simulink model "model2"  (R2023b)
settings: Solver=VariableStepAuto  StartTime=0.0  StopTime=8  RelTol=1e-3
values from neighbouring files (symbols this model uses):
  Bruitventx = 2    [dronecode.m]
  Bruitventy = 0.05    [dronecode.m]
  Consigneangle = pi/2    (= 1.570796327)    [dronecode.m]
  ConsigneVy = 0    [dronecode.m]
  Cx = 0.2    [dronecode.m]
  Freqfiltremoteur = 10    [dronecode.m]
  g = 9.81    [dronecode.m]
  J = 0.05    [dronecode.m]
  m = 0.9    [dronecode.m]
  pho = 1.225    [dronecode.m]
  Sref = 0.3    [dronecode.m]
libraries: simulink x9, cstblocks x3, embmathops x2, slpidlib x2, uavutilslib x1
settings Model: Creator=Utilisateur  LastModifiedBy=Utilisateur
settings SolverCC: ZeroCrossAlgorithm=Adaptive
settings OptimizationCC: ReuseModelBlockBuffer=off
settings DebuggingCC: IgnoredZcDiagnostic=none  UnconnectedInputMsg=warning  UnconnectedOutputMsg=warning  UnconnectedLineMsg=warning
settings ModelReferenceCC: EnableRefExpFcnMdlSchedulingChecks=on
settings RTWCC: DLArmComputeVersion=19.05

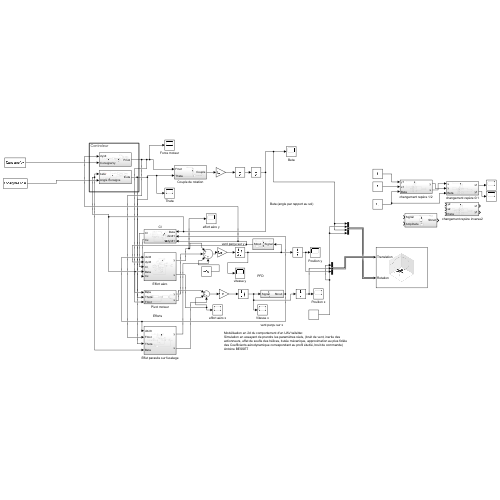
[thumbnail: Simulink's stored preview of the top-level diagram]
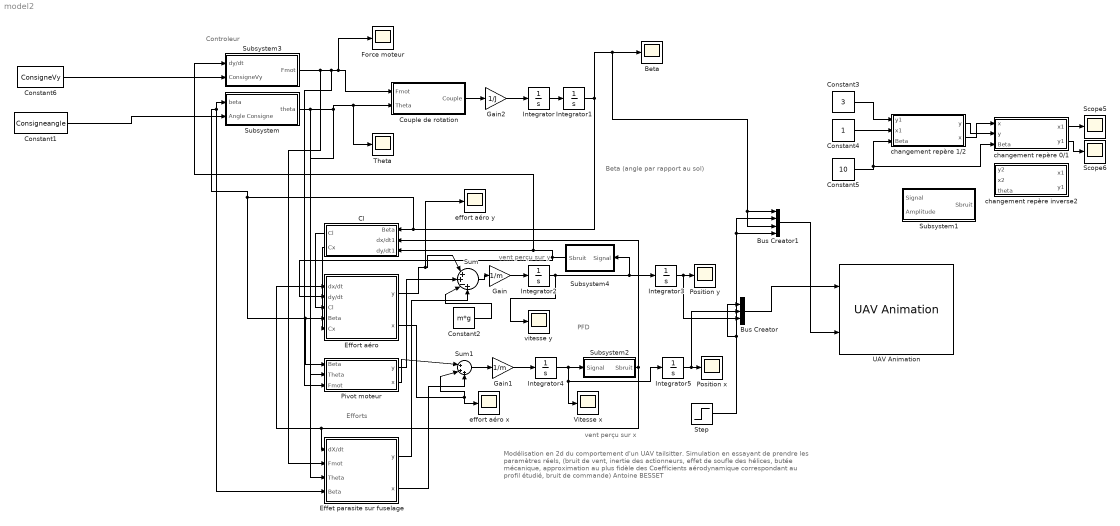
== system model2 ==
  note: vent perçu sur x
  note: Beta (angle par rapport au sol)
  note: Efforts
  note: PFD
  note: Controleur
  note: Modélisation en 2d du comportement d'un UAV tailsitter.
      | Simulation en essayant de prendre les paramètres réels, (bruit de vent, inertie des actionneurs, effet de soufle des hélices, butée mécanique, approximation au plus fidèle des Coefficients aérodynamique correspondant au profil étudié, bruit de commande)
      | Antoine BESSET
  note: vent perçu sur y
  Beta : Scope
  Bus Creator : BusCreator  Inputs=3
  Bus Creator1 : BusCreator  Inputs=4
  Cl : Subsystem
  Constant1 : Constant  Value=Consigneangle
  Constant2 : Constant  Value=m*g
  Constant3 : Constant  Value=3
  Constant4 : Constant
  Constant5 : Constant  Value=10
  Constant6 : Constant  Value=ConsigneVy
  Couple de rotation : Subsystem
  Effet parasite sur fuselage : Subsystem
  Effort aéro : Subsystem
  Force moteur : Scope
  Gain : Gain  Gain=1/m
  Gain1 : Gain  Gain=1/m
  Gain2 : Gain  Gain=1/J
  Integrator{,1,3,5} (4 alike) : Integrator
  Integrator2 : Integrator  LimitOutput=on  UpperSaturationLimit=100  LowerSaturationLimit=-100
  Integrator4 : Integrator  InitialCondition=10  LimitOutput=on  UpperSaturationLimit=100  LowerSaturationLimit=-100
  Pivot moteur : Subsystem
  Position x : Scope
  Position y : Scope
  Scope5 : Scope
  Scope6 : Scope
  Step : Step  Before=0.01  After=0.01  SampleTime=0
  Subsystem : Subsystem
  Subsystem1 : Subsystem
  Subsystem2 : Subsystem
  Subsystem3 : Subsystem
  Subsystem4 : Subsystem
  Sum : Sum  Inputs=|++-+
  Sum1 : Sum  Inputs=|+++
  Theta : Scope
  UAV Animation : uavutilslib/UAV Animation  UAVType=FixedWing  UAVSize=1  InertialZDirection=Up  SampleTime=-1
  Vitesse x : Scope
  changement repère 0/1 : Subsystem
  changement repère 1/2 : Subsystem
  changement repère inverse2 : Subsystem
  effort aéro x : Scope
  effort aéro y : Scope
  vitesse y : Scope
  wires:
  Subsystem/1(theta) -> Pivot moteur/2(Theta), Theta/1, Couple de rotation/2(Theta), Effet parasite sur fuselage/3(Theta)
  Integrator/1 -> Integrator1/1
  Cl/1(Cl) -> Effort aéro/3(Cl)
  Pivot moteur/1(y) -> Sum/2
  Constant2/1 -> Sum/3
  Pivot moteur/2(x) -> Sum1/1
  Effort aéro/2(x) -> effort aéro x/1, Sum1/2
  Gain1/1 -> Integrator4/1
  Sum1/1 -> Gain1/1
  Sum/1 -> Gain/1
  Gain/1 -> Integrator2/1
  Integrator4/1 -> Integrator5/1, Vitesse x/1, Subsystem2/1(Signal)
  Integrator5/1 -> Bus Creator/2, Position x/1
  Integrator2/1 -> Integrator3/1, Subsystem4/1(Signal), vitesse y/1
  Effort aéro/1(y) -> effort aéro y/1, Sum/1
  changement repère 1/2/2(x) -> changement repère 0/1/1(x)
  changement repère 1/2/1(y) -> changement repère 0/1/2(y)
  Constant5/1 -> changement repère 0/1/3(Beta), changement repère 1/2/3(Beta)
  Constant4/1 -> changement repère 1/2/2(x1)
  Constant3/1 -> changement repère 1/2/1(y1)
  changement repère 0/1/1(x1) -> Scope5/1
  changement repère 0/1/2(y1) -> Scope6/1
  Cl/2(Cx) -> Effort aéro/5(Cx)
  Couple de rotation/1(Couple) -> Gain2/1
  Gain2/1 -> Integrator/1
  Subsystem2/1(Sbruit) -> Cl/2(dx/dt1), Effet parasite sur fuselage/1(dX/dt), Effort aéro/1(dx/dt)
  Subsystem4/1(Sbruit) -> Subsystem3/1(dy/dt), Cl/3(dy/dt1), Effort aéro/2(dy/dt)
  Subsystem3/1(Fmot) -> Effet parasite sur fuselage/2(Fmot), Pivot moteur/3(Fmot), Force moteur/1, Couple de rotation/1(Fmot)
  Effet parasite sur fuselage/2(x) -> Sum1/3
  Effet parasite sur fuselage/1(y) -> Sum/4
  Constant6/1 -> Subsystem3/2(ConsigneVy)
  Constant1/1 -> Subsystem/2(Angle Consigne)
  Bus Creator/1 -> UAV Animation/1
  Step/1 -> Bus Creator1/4, Bus Creator1/2, Bus Creator/1
  Bus Creator1/1 -> UAV Animation/2
  Integrator3/1 -> Bus Creator/3, Position y/1
  Integrator1/1 -> Effet parasite sur fuselage/4(Beta), Subsystem/1(beta), Pivot moteur/1(Beta), Effort aéro/4(Beta), Cl/1(Beta), Bus Creator1/1, Bus Creator1/3, Beta/1

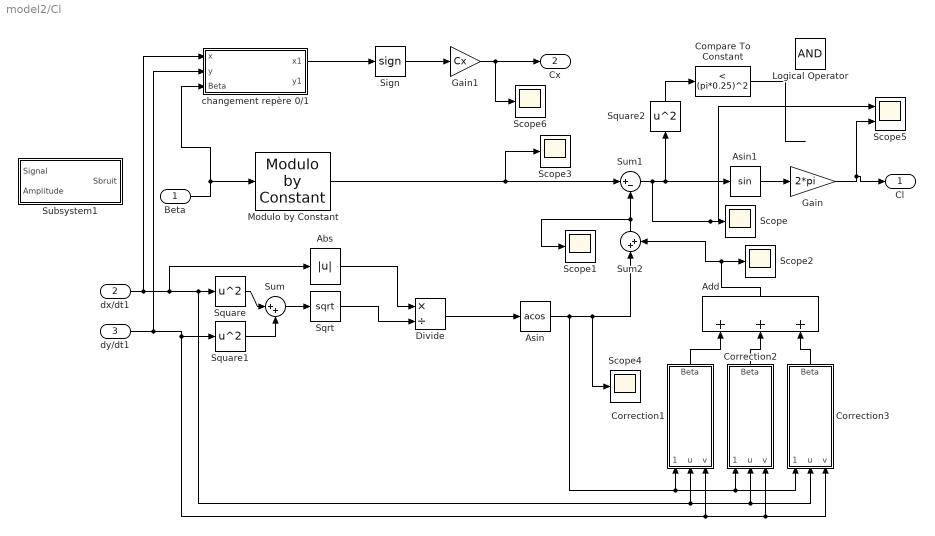
== system model2/Cl ==
  Beta : Inport
  dx/dt1 : Inport  Port=2
  dy/dt1 : Inport  Port=3
  Abs : Abs  SaturateOnIntegerOverflow=off
  Add : Sum  Inputs=+++
  Asin : Trigonometry  Operator=acos  OutputSignalType=real
  Asin1 : Trigonometry
  Compare To Constant : simulink/Logic and Bit Operations/Compare To Constant  relop=<  const=(pi*0.25)^2  OutDataTypeStr=boolean
  Correction1 : Subsystem
  Correction2 : Subsystem
  Correction3 : Subsystem
  Divide : Product  Inputs=*/
  Gain : Gain  Gain=2*pi
  Gain1 : Gain  Gain=Cx
  Logical Operator : Logic  AllPortsSameDT=off  OutDataTypeStr=boolean
  Modulo by Constant : embmathops/Modulo by Constant  Denominator=2*pi  SimulateUsing=Code generation
  Scope{,1..4,6} (6 alike) : Scope
  Scope5 : Scope  NumInputPorts=2
  Sign : Signum
  Sqrt : Sqrt
  Square : Math  Operator=square
  Square1 : Math  Operator=square
  Square2 : Math  Operator=square
  Subsystem1 : Subsystem
  Sum : Sum  Inputs=|++
  Sum1 : Sum  Inputs=|+-
  Sum2 : Sum  Inputs=|++
  changement repère 0/1 : Subsystem
  Cl : Outport
  Cx : Outport  Port=2
  wires:
  dy/dt1/1 -> changement repère 0/1/2(y), Correction3/3(v), Correction2/3(v), Correction1/3(v), Square1/1
  Square/1 -> Sum/1
  dx/dt1/1 -> changement repère 0/1/1(x), Correction3/2(u), Correction2/2(u), Correction1/2(u), Square/1, Abs/1
  Square1/1 -> Sum/2
  Sum/1 -> Sqrt/1
  Sqrt/1 -> Divide/2
  Divide/1 -> Asin/1
  Beta/1 -> changement repère 0/1/3(Beta), Modulo by Constant/1
  Modulo by Constant/1 -> Scope3/1, Sum1/1
  Abs/1 -> Divide/1
  Asin/1 -> Correction3/1(theta), Correction2/1(theta), Correction1/1(theta), Scope4/1, Sum2/1
  Add/1 -> Sum2/2, Scope2/1
  Correction1/1(Beta) -> Add/1
  Correction2/1(Beta) -> Add/2
  Correction3/1(Beta) -> Add/3
  Asin1/1 -> Gain/1
  Gain1/1 -> Scope6/1, Cx/1
  Sum2/1 -> Scope1/1, Sum1/2
  Sign/1 -> Gain1/1
  changement repère 0/1/1(x1) -> Sign/1
  Square2/1 -> Compare To Constant/1
  Gain/1 -> Scope5/2, Cl/1
  Compare To Constant/1 -> ?
  Sum1/1 -> Scope5/1, Scope/1, Asin1/1, Square2/1

== system model2/Couple de rotation ==
  Fmot : Inport
  Theta : Inport  Port=2
  Gain : Gain  Gain=0.10
  Product2 : Product
  Trigonometric Function : Trigonometry
  Couple : Outport
  wires:
  Theta/1 -> Trigonometric Function/1
  Fmot/1 -> Product2/2
  Trigonometric Function/1 -> Gain/1
  Product2/1 -> Couple/1
  Gain/1 -> Product2/1

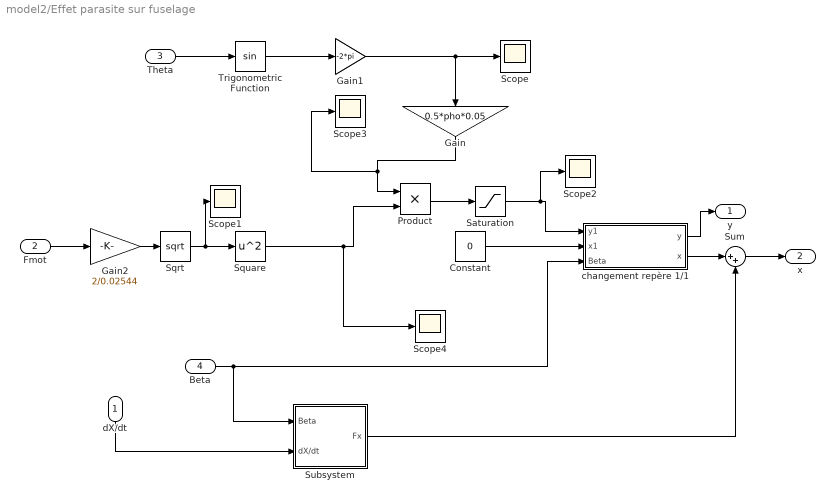
== system model2/Effet parasite sur fuselage ==
  dX/dt : Inport
  Fmot : Inport  Port=2
  Theta : Inport  Port=3
  Beta : Inport  Port=4
  Constant : Constant  Value=0
  Gain : Gain  Gain=0.5*pho*0.05
  Gain1 : Gain  Gain=-2*pi
  Gain2 : Gain  Gain=2/0.02544
  Product : Product
  Saturation : Saturate  UpperLimit=20  LowerLimit=-20
  Scope{,1..4} (5 alike) : Scope
  Sqrt : Sqrt
  Square : Math  Operator=square
  Subsystem : Subsystem
  Sum : Sum  Inputs=|++
  Trigonometric Function : Trigonometry
  changement repère 1/1 : Subsystem
  y : Outport
  x : Outport  Port=2
  wires:
  Square/1 -> Scope4/1, Product/2
  Gain/1 -> Scope3/1, Product/1
  Beta/1 -> Subsystem/1(Beta), changement repère 1/1/3(Beta)
  changement repère 1/1/1(y) -> y/1
  Gain1/1 -> Scope/1, Gain/1
  Gain2/1 -> Sqrt/1
  Fmot/1 -> Gain2/1
  Sqrt/1 -> Scope1/1, Square/1
  Constant/1 -> changement repère 1/1/2(x1)
  Theta/1 -> Trigonometric Function/1
  Trigonometric Function/1 -> Gain1/1
  Product/1 -> Saturation/1
  Saturation/1 -> Scope2/1, changement repère 1/1/1(y1)
  dX/dt/1 -> Subsystem/2(dX/dt)
  changement repère 1/1/2(x) -> Sum/1
  Sum/1 -> x/1
  Subsystem/1(Fx) -> Sum/2

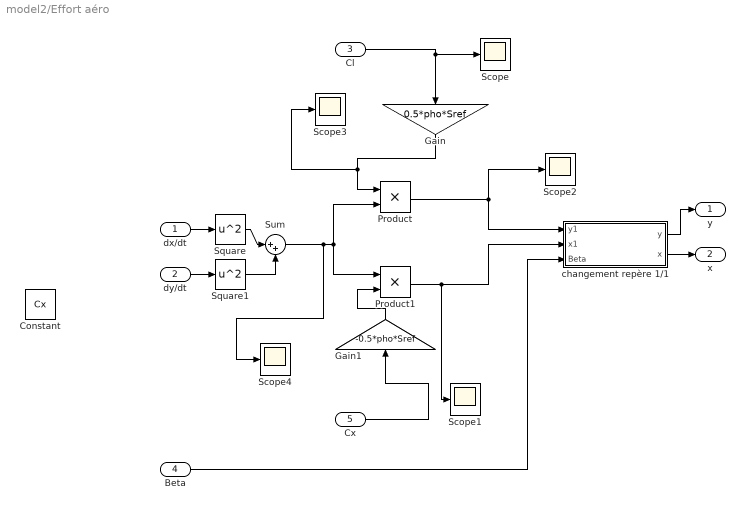
== system model2/Effort aéro ==
  dx/dt : Inport
  dy/dt : Inport  Port=2
  Cl : Inport  Port=3
  Beta : Inport  Port=4
  Cx : Inport  Port=5
  Constant : Constant  Value=Cx
  Gain : Gain  Gain=0.5*pho*Sref
  Gain1 : Gain  Gain=-0.5*pho*Sref
  Product : Product
  Product1 : Product
  Scope{,1..4} (5 alike) : Scope
  Square : Math  Operator=square
  Square1 : Math  Operator=square
  Sum : Sum  Inputs=|++
  changement repère 1/1 : Subsystem
  y : Outport
  x : Outport  Port=2
  wires:
  dx/dt/1 -> Square/1
  dy/dt/1 -> Square1/1
  Square1/1 -> Sum/2
  Square/1 -> Sum/1
  Sum/1 -> Scope4/1, Product1/1, Product/2
  Cl/1 -> Scope/1, Gain/1
  Gain/1 -> Scope3/1, Product/1
  Gain1/1 -> Product1/2
  Product/1 -> changement repère 1/1/1(y1), Scope2/1
  Product1/1 -> Scope1/1, changement repère 1/1/2(x1)
  Beta/1 -> changement repère 1/1/3(Beta)
  changement repère 1/1/2(x) -> x/1
  changement repère 1/1/1(y) -> y/1
  Cx/1 -> Gain1/1

== system model2/Pivot moteur ==
  Beta : Inport
  Theta : Inport  Port=2
  Fmot : Inport  Port=3
  Constant : Constant  Value=0
  changement repère 1/1 : Subsystem
  changement repère inverse2/1 : Subsystem
  y : Outport
  x : Outport  Port=2
  wires:
  Theta/1 -> changement repère inverse2/1/3(theta)
  Fmot/1 -> changement repère inverse2/1/2(x2)
  changement repère inverse2/1/2(y1) -> changement repère 1/1/1(y1)
  changement repère inverse2/1/1(x1) -> changement repère 1/1/2(x1)
  changement repère 1/1/2(x) -> x/1
  changement repère 1/1/1(y) -> y/1
  Constant/1 -> changement repère inverse2/1/1(y2)
  Beta/1 -> changement repère 1/1/3(Beta)

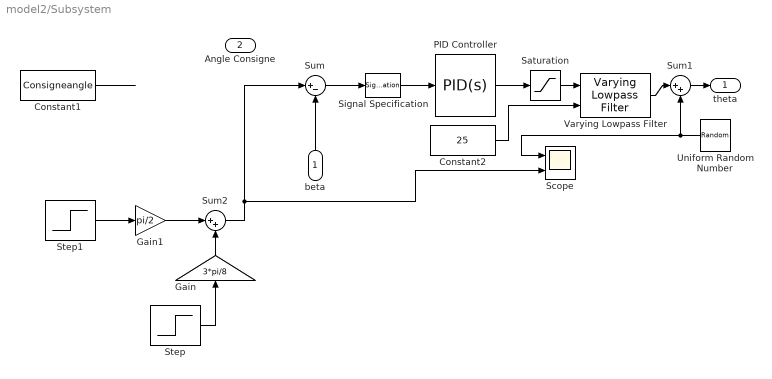
== system model2/Subsystem ==
  beta : Inport
  Angle Consigne : Inport  Port=2
  Constant1 : Constant  Value=Consigneangle
  Constant2 : Constant  Value=25
  Gain : Gain  Gain=3*pi/8
  Gain1 : Gain  Gain=pi/2
  PID Controller : slpidlib/PID Controller  Controller=PID  Form=Parallel  TimeDomain=Continuous-time  UseExternalTs=off  SampleTime=-1  IntegratorMethod=Forward Euler  FilterMethod=Forward Euler  ControllerParametersSource=internal  P=1  I=0.3  UseKiTs=off  D=0.5  N=100  UseFilter=on  TunerSelectOption=Transfer Function Based (PID Tuner App)  InitialConditionSource=internal  InitialConditionForIntegrator=0  InitialConditionForFilter=0  DifferentiatorICPrevScaledInput=0  ExternalReset=none  TrackingMode=off  Kt=1  LimitOutput=on  SatLimitsSource=internal  UpperSaturationLimit=pi/4  LowerSaturationLimit=-pi/4  LinearizeAsGain=on  AntiWindupMode=none  Kb=1  LimitIntegrator=off  UpperIntegratorSaturationLimit=inf  LowerIntegratorSaturationLimit=-inf  POutMin=[]  POutMax=[]  IOutMin=[]  IOutMax=[]  DOutMin=[]  DOutMax=[]  NOutMin=[]  NOutMax=[]  SumOutMin=[]  SumOutMax=[]  SaturationOutMin=[]  SaturationOutMax=[]  PParamMin=[]  PParamMax=[]  IParamMin=[]  IParamMax=[]  DParamMin=[]  DParamMax=[]  NParamMin=[]  NParamMax=[]  KbParamMin=[]  KbParamMax=[]  KtParamMin=[]  KtParamMax=[]  KbOutMin=[]  KbOutMax=[]  KtOutMin=[]  KtOutMax=[]  IntegratorOutMin=[]  IntegratorOutMax=[]  FilterOutMin=[]  FilterOutMax=[]  SumI1OutMin=[]  SumI1OutMax=[]  SumI2OutMin=[]  SumI2OutMax=[]  SumI3OutMin=[]  SumI3OutMax=[]  SumI4OutMin=[]  SumI4OutMax=[]  SumDOutMin=[]  SumDOutMax=[]  DifferentiatorOutMin=[]  DifferentiatorOutMax=[]  FilterDiffOutCoefMin=[]  FilterDiffOutCoefMax=[]  ReciprocalOutMin=[]  ReciprocalOutMax=[]  SumDenOutMin=[]  SumDenOutMax=[]  SumNumOutMin=[]  SumNumOutMax=[]  DivideOutMin=[]  DivideOutMax=[]  UdiffTsProdOutMin=[]  UdiffTsProdOutMax=[]  NTsProdOutMin=[]  NTsProdOutMax=[]  UintegralTsProdOutMin=[]  UintegralTsProdOutMax=[]  UngainTsProdOutMin=[]  UngainTsProdOutMax=[]  ClampingZeroOutDataTypeStr=Inherit: Inherit via back propagation  ClampingZeroOutMin=[]  ClampingZeroOutMax=[]  FilterDenConstantOutDataTypeStr=Inherit: Inherit via back propagation  FilterDenConstantOutMin=[]  FilterDenConstantOutMax=[]  PCopyOutDataTypeStr=Inherit: Inherit via back propagation  PCopyOutMin=[]  PCopyOutMax=[]  NCopyOutDataTypeStr=Inherit: Inherit via back propagation  NCopyOutMin=[]  NCopyOutMax=[]  IntegratorContinuousStateAttributes=''  IntegratorStateMustResolveToSignalObject=off  IntegratorRTWStateStorageClass=Auto  FilterContinuousStateAttributes=''  FilterStateMustResolveToSignalObject=off  FilterRTWStateStorageClass=Auto  ParallelPVariant=InternalParameters  IdealPVariant=Disabled  IVariant=InternalParameters  DVariant=InternalParameters  IntegratorVariant=Continuous  SatVariant=Enabled  AWVariant=Passthrough  PCopyVariant=Disabled  TRVariant=Disabled  FdbkBlocksVariant=Forward  IdealPFdbkVariant=Disabled  SatFdbkVariant=Disabled  DerivativeFilterVariant=ContFilter  NVariant=InternalParameters  NCopyVariant=Disabled  FilterICVariant=InternalICsFilter  IntegratorICVariant=InternalICs  ExternalResetVariant=Disabled  TRSumVariant=Passthrough  SumFdbkVariant=Disabled  SumVariant=Sum_PID  TsampFilterVariant=InternalTs  TsampNgainVariant=Passthrough  TsampIntegralVariant=Disabled_SignalSpec  ExternalSaturationOutDataTypeStr=Inherit: Same as second input
  Saturation : Saturate  UpperLimit=pi/4  LowerLimit=-pi/4
  Scope : Scope  NumInputPorts=2
  Signal Specification : SignalSpecification  Dimensions=1
  Step : Step  Time=5  After=-1  SampleTime=0
  Step1 : Step  Before=0.1  SampleTime=0
  Sum : Sum  Inputs=|+-
  Sum1 : Sum  Inputs=|++
  Sum2 : Sum  Inputs=|++
  Uniform Random Number : UniformRandomNumber  Minimum=-0.05  Maximum=0.05  SampleTime=0.01
  Varying Lowpass Filter : cstblocks/Linear Parameter Varying/Varying Lowpass Filter  N=1
  theta : Outport
  wires:
  beta/1 -> Sum/2
  Sum1/1 -> theta/1
  Uniform Random Number/1 -> Scope/1, Sum1/2
  Signal Specification/1 -> PID Controller/1
  Sum/1 -> Signal Specification/1
  Gain/1 -> Sum2/2
  Step/1 -> Gain/1
  Gain1/1 -> Sum2/1
  Step1/1 -> Gain1/1
  PID Controller/1 -> Saturation/1
  Saturation/1 -> Varying Lowpass Filter/1
  Varying Lowpass Filter/1 -> Sum1/1
  Constant2/1 -> Varying Lowpass Filter/2
  Constant1/1 -> ?
  Sum2/1 -> Sum/1, Scope/2

== system model2/Subsystem1 ==
  Signal : Inport
  Amplitude : Inport  Port=2
  Product : Product
  Sum2 : Sum  Inputs=|++
  Uniform Random Number : UniformRandomNumber  SampleTime=0.01
  Sbruit : Outport
  wires:
  Signal/1 -> Sum2/1
  Sum2/1 -> Sbruit/1
  Uniform Random Number/1 -> Product/2
  Product/1 -> Sum2/2
  Amplitude/1 -> Product/1

== system model2/Subsystem2 ==
  Signal : Inport
  Constant : Constant  Value=Bruitventx
  Constant2 : Constant
  Product : Product
  Scope : Scope
  Sum2 : Sum  Inputs=|++
  Uniform Random Number : UniformRandomNumber  Minimum=-10  Maximum=10  SampleTime=0.01
  Varying Lowpass Filter1 : cstblocks/Linear Parameter Varying/Varying Lowpass Filter  N=1
  Sbruit : Outport
  wires:
  Signal/1 -> Sum2/1
  Uniform Random Number/1 -> Product/2
  Constant/1 -> Product/1
  Sum2/1 -> Sbruit/1
  Constant2/1 -> Varying Lowpass Filter1/2
  Product/1 -> Varying Lowpass Filter1/1
  Varying Lowpass Filter1/1 -> Scope/1, Sum2/2

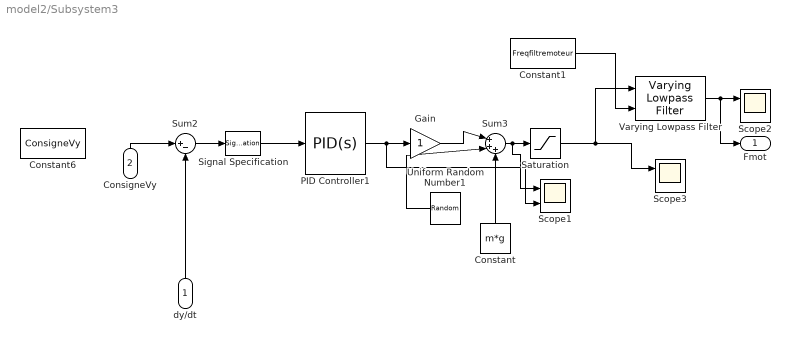
== system model2/Subsystem3 ==
  dy/dt : Inport
  ConsigneVy : Inport  Port=2
  Constant : Constant  Value=m*g
  Constant1 : Constant  Value=Freqfiltremoteur
  Constant6 : Constant  Value=ConsigneVy
  Gain : Gain
  PID Controller1 : slpidlib/PID Controller  Controller=PID  Form=Parallel  TimeDomain=Continuous-time  UseExternalTs=off  SampleTime=0.1  IntegratorMethod=Forward Euler  FilterMethod=Forward Euler  ControllerParametersSource=internal  P=1.2  I=0.6  UseKiTs=off  D=0.2  N=100  UseFilter=on  TunerSelectOption=Transfer Function Based (PID Tuner App)  InitialConditionSource=internal  InitialConditionForIntegrator=0  InitialConditionForFilter=0  DifferentiatorICPrevScaledInput=0  ExternalReset=none  TrackingMode=off  Kt=1  LimitOutput=off  SatLimitsSource=internal  UpperSaturationLimit=inf  LowerSaturationLimit=-inf  LinearizeAsGain=on  AntiWindupMode=none  Kb=1  LimitIntegrator=off  UpperIntegratorSaturationLimit=inf  LowerIntegratorSaturationLimit=-inf  POutMin=[]  POutMax=[]  IOutMin=[]  IOutMax=[]  DOutMin=[]  DOutMax=[]  NOutMin=[]  NOutMax=[]  SumOutMin=[]  SumOutMax=[]  SaturationOutMin=[]  SaturationOutMax=[]  PParamMin=[]  PParamMax=[]  IParamMin=[]  IParamMax=[]  DParamMin=[]  DParamMax=[]  NParamMin=[]  NParamMax=[]  KbParamMin=[]  KbParamMax=[]  KtParamMin=[]  KtParamMax=[]  KbOutMin=[]  KbOutMax=[]  KtOutMin=[]  KtOutMax=[]  IntegratorOutMin=[]  IntegratorOutMax=[]  FilterOutMin=[]  FilterOutMax=[]  SumI1OutMin=[]  SumI1OutMax=[]  SumI2OutMin=[]  SumI2OutMax=[]  SumI3OutMin=[]  SumI3OutMax=[]  SumI4OutMin=[]  SumI4OutMax=[]  SumDOutMin=[]  SumDOutMax=[]  DifferentiatorOutMin=[]  DifferentiatorOutMax=[]  FilterDiffOutCoefMin=[]  FilterDiffOutCoefMax=[]  ReciprocalOutMin=[]  ReciprocalOutMax=[]  SumDenOutMin=[]  SumDenOutMax=[]  SumNumOutMin=[]  SumNumOutMax=[]  DivideOutMin=[]  DivideOutMax=[]  UdiffTsProdOutMin=[]  UdiffTsProdOutMax=[]  NTsProdOutMin=[]  NTsProdOutMax=[]  UintegralTsProdOutMin=[]  UintegralTsProdOutMax=[]  UngainTsProdOutMin=[]  UngainTsProdOutMax=[]  ClampingZeroOutDataTypeStr=Inherit: Inherit via back propagation  ClampingZeroOutMin=[]  ClampingZeroOutMax=[]  FilterDenConstantOutDataTypeStr=Inherit: Inherit via back propagation  FilterDenConstantOutMin=[]  FilterDenConstantOutMax=[]  PCopyOutDataTypeStr=Inherit: Inherit via back propagation  PCopyOutMin=[]  PCopyOutMax=[]  NCopyOutDataTypeStr=Inherit: Inherit via back propagation  NCopyOutMin=[]  NCopyOutMax=[]  IntegratorContinuousStateAttributes=''  IntegratorStateMustResolveToSignalObject=off  IntegratorRTWStateStorageClass=Auto  FilterContinuousStateAttributes=''  FilterStateMustResolveToSignalObject=off  FilterRTWStateStorageClass=Auto  ParallelPVariant=InternalParameters  IdealPVariant=Disabled  IVariant=InternalParameters  DVariant=InternalParameters  IntegratorVariant=Continuous  SatVariant=Disabled  AWVariant=Passthrough  PCopyVariant=Disabled  TRVariant=Disabled  FdbkBlocksVariant=Forward  IdealPFdbkVariant=Disabled  SatFdbkVariant=Disabled  DerivativeFilterVariant=ContFilter  NVariant=InternalParameters  NCopyVariant=Disabled  FilterICVariant=InternalICsFilter  IntegratorICVariant=InternalICs  ExternalResetVariant=Disabled  TRSumVariant=Passthrough  SumFdbkVariant=Disabled  SumVariant=Sum_PID  TsampFilterVariant=InternalTs  TsampNgainVariant=Passthrough  TsampIntegralVariant=Disabled_SignalSpec  ExternalSaturationOutDataTypeStr=Inherit: Same as second input
  Saturation : Saturate  UpperLimit=40  LowerLimit=0
  Scope1 : Scope  NumInputPorts=2
  Scope2 : Scope  NumInputPorts=2
  Scope3 : Scope  NumInputPorts=2
  Signal Specification : SignalSpecification  Dimensions=1
  Sum2 : Sum  Inputs=|+-
  Sum3 : Sum  Inputs=|+++
  Uniform Random Number1 : UniformRandomNumber  Minimum=-0.01  Maximum=0.01  SampleTime=0.01
  Varying Lowpass Filter : cstblocks/Linear Parameter Varying/Varying Lowpass Filter  N=1
  Fmot : Outport
  wires:
  Saturation/1 -> Varying Lowpass Filter/1, Scope3/1
  dy/dt/1 -> Sum2/2
  Sum3/1 -> Scope1/1, Saturation/1
  Uniform Random Number1/1 -> Sum3/2
  PID Controller1/1 -> Gain/1, Scope1/2
  Constant/1 -> Sum3/3
  Gain/1 -> Sum3/1
  Sum2/1 -> Signal Specification/1
  Signal Specification/1 -> PID Controller1/1
  Varying Lowpass Filter/1 -> Fmot/1, Scope2/1
  Constant1/1 -> Varying Lowpass Filter/2
  ConsigneVy/1 -> Sum2/1

== system model2/Subsystem4 ==
  Signal : Inport
  Constant1 : Constant  Value=Bruitventy
  Product : Product
  Sum2 : Sum  Inputs=|++
  Uniform Random Number : UniformRandomNumber  SampleTime=0.01
  Sbruit : Outport
  wires:
  Signal/1 -> Sum2/1
  Sum2/1 -> Sbruit/1
  Uniform Random Number/1 -> Product/2
  Product/1 -> Sum2/2
  Constant1/1 -> Product/1

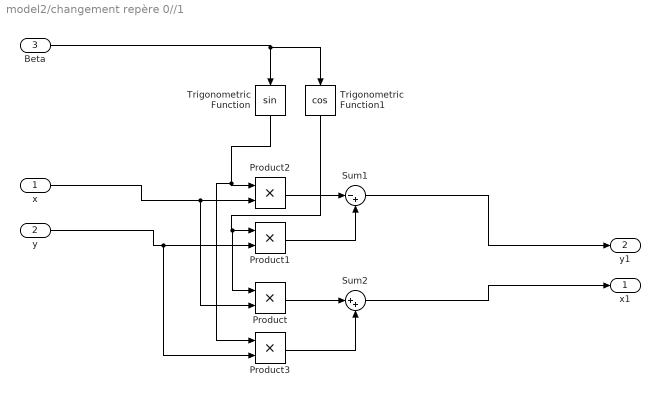
== system model2/changement repère 0//1 ==
  x : Inport
  y : Inport  Port=2
  Beta : Inport  Port=3
  Product{,1..3} (4 alike) : Product
  Sum1 : Sum  Inputs=|-+
  Sum2 : Sum  Inputs=|++
  Trigonometric Function : Trigonometry
  Trigonometric Function1 : Trigonometry  Operator=cos
  x1 : Outport
  y1 : Outport  Port=2
  wires:
  Beta/1 -> Trigonometric Function1/1, Trigonometric Function/1
  Trigonometric Function/1 -> Product3/1, Product2/1
  Product2/1 -> Sum1/1
  x/1 -> Product/2, Product2/2
  y/1 -> Product3/2, Product1/2
  Trigonometric Function1/1 -> Product/1, Product1/1
  Product1/1 -> Sum1/2
  Sum1/1 -> y1/1
  Product3/1 -> Sum2/2
  Product/1 -> Sum2/1
  Sum2/1 -> x1/1

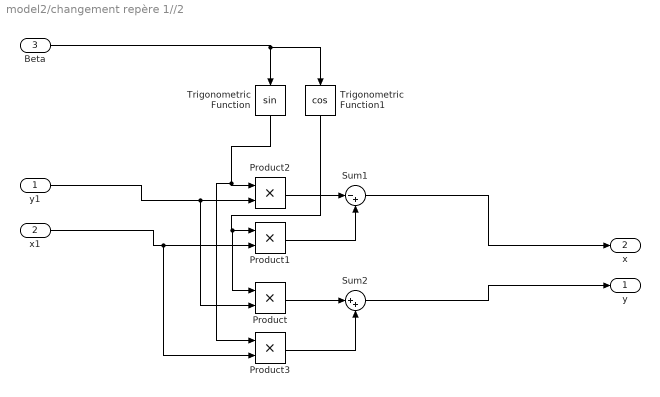
== system model2/changement repère 1//2 ==
  y1 : Inport
  x1 : Inport  Port=2
  Beta : Inport  Port=3
  Product{,1..3} (4 alike) : Product
  Sum1 : Sum  Inputs=|-+
  Sum2 : Sum  Inputs=|++
  Trigonometric Function : Trigonometry
  Trigonometric Function1 : Trigonometry  Operator=cos
  y : Outport
  x : Outport  Port=2
  wires:
  Beta/1 -> Trigonometric Function1/1, Trigonometric Function/1
  Trigonometric Function/1 -> Product3/1, Product2/1
  Product2/1 -> Sum1/1
  y1/1 -> Product/2, Product2/2
  x1/1 -> Product3/2, Product1/2
  Trigonometric Function1/1 -> Product/1, Product1/1
  Product1/1 -> Sum1/2
  Sum1/1 -> x/1
  Product3/1 -> Sum2/2
  Product/1 -> Sum2/1
  Sum2/1 -> y/1

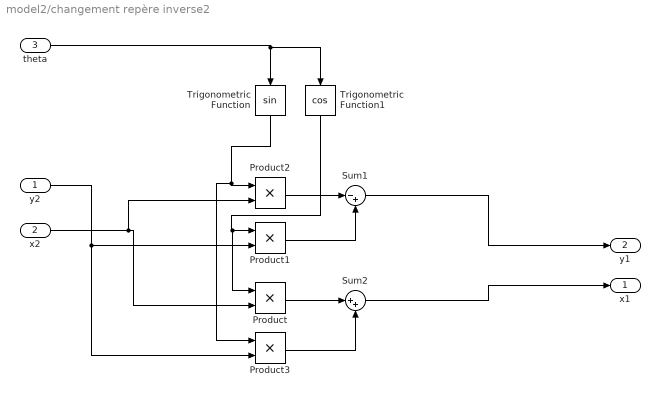
== system model2/changement repère inverse2 ==
  y2 : Inport
  x2 : Inport  Port=2
  theta : Inport  Port=3
  Product{,1..3} (4 alike) : Product
  Sum1 : Sum  Inputs=|-+
  Sum2 : Sum  Inputs=|++
  Trigonometric Function : Trigonometry
  Trigonometric Function1 : Trigonometry  Operator=cos
  x1 : Outport
  y1 : Outport  Port=2
  wires:
  theta/1 -> Trigonometric Function1/1, Trigonometric Function/1
  Trigonometric Function/1 -> Product3/1, Product2/1
  Product2/1 -> Sum1/1
  Trigonometric Function1/1 -> Product/1, Product1/1
  Product1/1 -> Sum1/2
  Sum1/1 -> y1/1
  Product3/1 -> Sum2/2
  Product/1 -> Sum2/1
  Sum2/1 -> x1/1
  x2/1 -> Product2/2, Product/2
  y2/1 -> Product1/2, Product3/2

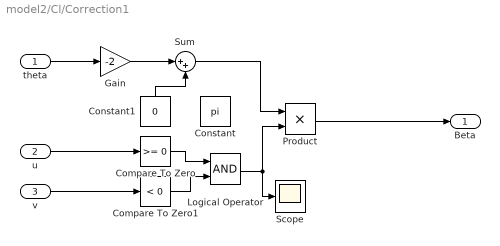
== system model2/Cl/Correction1 ==
  theta : Inport
  u : Inport  Port=2
  v : Inport  Port=3
  Compare To Zero : simulink/Logic and Bit Operations/Compare To Zero  relop=>=  OutDataTypeStr=boolean
  Compare To Zero1 : simulink/Logic and Bit Operations/Compare To Zero  relop=<  OutDataTypeStr=boolean
  Constant : Constant  Value=pi
  Constant1 : Constant  Value=0
  Gain : Gain  Gain=-2
  Logical Operator : Logic  AllPortsSameDT=off  OutDataTypeStr=boolean
  Product : Product
  Scope : Scope
  Sum : Sum  Inputs=|++
  Beta : Outport
  wires:
  u/1 -> Compare To Zero/1
  v/1 -> Compare To Zero1/1
  Compare To Zero/1 -> Logical Operator/1
  Compare To Zero1/1 -> Logical Operator/2
  Product/1 -> Beta/1
  Sum/1 -> Product/1
  theta/1 -> Gain/1
  Gain/1 -> Sum/1
  Constant1/1 -> Sum/2
  Logical Operator/1 -> Product/2, Scope/1

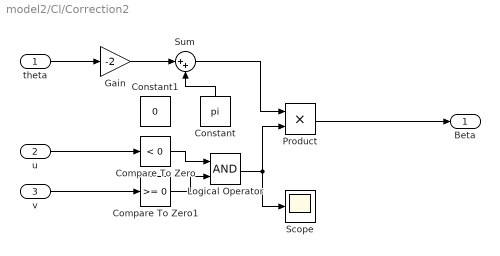
== system model2/Cl/Correction2 ==
  theta : Inport
  u : Inport  Port=2
  v : Inport  Port=3
  Compare To Zero : simulink/Logic and Bit Operations/Compare To Zero  relop=<  OutDataTypeStr=boolean
  Compare To Zero1 : simulink/Logic and Bit Operations/Compare To Zero  relop=>=  OutDataTypeStr=boolean
  Constant : Constant  Value=pi
  Constant1 : Constant  Value=0
  Gain : Gain  Gain=-2
  Logical Operator : Logic  AllPortsSameDT=off  OutDataTypeStr=boolean
  Product : Product
  Scope : Scope
  Sum : Sum  Inputs=|++
  Beta : Outport
  wires:
  u/1 -> Compare To Zero/1
  v/1 -> Compare To Zero1/1
  Compare To Zero/1 -> Logical Operator/1
  Compare To Zero1/1 -> Logical Operator/2
  Logical Operator/1 -> Product/2, Scope/1
  Product/1 -> Beta/1
  Sum/1 -> Product/1
  theta/1 -> Gain/1
  Gain/1 -> Sum/1
  Constant/1 -> Sum/2

== system model2/Cl/Correction3 ==
  theta : Inport
  u : Inport  Port=2
  v : Inport  Port=3
  Compare To Zero : simulink/Logic and Bit Operations/Compare To Zero  relop=<  OutDataTypeStr=boolean
  Compare To Zero1 : simulink/Logic and Bit Operations/Compare To Zero  relop=<  OutDataTypeStr=boolean
  Constant : Constant  Value=pi
  Constant1 : Constant  Value=0
  Gain : Gain  Gain=0
  Logical Operator : Logic  AllPortsSameDT=off  OutDataTypeStr=boolean
  Product : Product
  Scope : Scope
  Sum : Sum  Inputs=|++
  Beta : Outport
  wires:
  u/1 -> Compare To Zero/1
  v/1 -> Compare To Zero1/1
  Compare To Zero/1 -> Logical Operator/1
  Compare To Zero1/1 -> Logical Operator/2
  Logical Operator/1 -> Product/2, Scope/1
  Product/1 -> Beta/1
  Sum/1 -> Product/1
  theta/1 -> Gain/1
  Gain/1 -> Sum/1
  Constant/1 -> Sum/2

== system model2/Cl/Subsystem1 ==
  Signal : Inport
  Amplitude : Inport  Port=2
  Product : Product
  Sum2 : Sum  Inputs=|++
  Uniform Random Number : UniformRandomNumber  SampleTime=0.01
  Sbruit : Outport
  wires:
  Signal/1 -> Sum2/1
  Sum2/1 -> Sbruit/1
  Uniform Random Number/1 -> Product/2
  Product/1 -> Sum2/2
  Amplitude/1 -> Product/1

== system model2/Cl/changement repère 0//1 ==
  x : Inport
  y : Inport  Port=2
  Beta : Inport  Port=3
  Product{,1..3} (4 alike) : Product
  Sum1 : Sum  Inputs=|-+
  Sum2 : Sum  Inputs=|++
  Trigonometric Function : Trigonometry
  Trigonometric Function1 : Trigonometry  Operator=cos
  x1 : Outport
  y1 : Outport  Port=2
  wires:
  Beta/1 -> Trigonometric Function1/1, Trigonometric Function/1
  Trigonometric Function/1 -> Product3/1, Product2/1
  Product2/1 -> Sum1/1
  x/1 -> Product/2, Product2/2
  y/1 -> Product3/2, Product1/2
  Trigonometric Function1/1 -> Product/1, Product1/1
  Product1/1 -> Sum1/2
  Sum1/1 -> y1/1
  Product3/1 -> Sum2/2
  Product/1 -> Sum2/1
  Sum2/1 -> x1/1

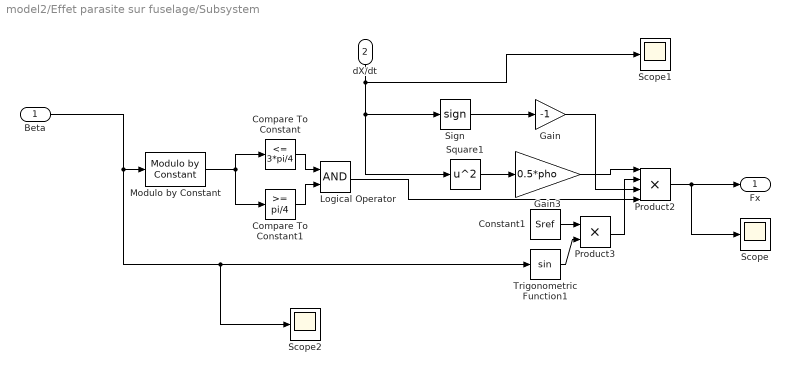
== system model2/Effet parasite sur fuselage/Subsystem ==
  Beta : Inport
  dX/dt : Inport  Port=2
  Compare To Constant : simulink/Logic and Bit Operations/Compare To Constant  relop=<=  const=3*pi/4  OutDataTypeStr=boolean
  Compare To Constant1 : simulink/Logic and Bit Operations/Compare To Constant  relop=>=  const=pi/4  OutDataTypeStr=boolean
  Constant1 : Constant  Value=Sref
  Gain : Gain  Gain=-1
  Gain3 : Gain  Gain=0.5*pho
  Logical Operator : Logic  AllPortsSameDT=off  OutDataTypeStr=boolean
  Modulo by Constant : embmathops/Modulo by Constant  Denominator=2*pi  SimulateUsing=Code generation
  Product2 : Product  Inputs=4
  Product3 : Product
  Scope : Scope
  Scope1 : Scope
  Scope2 : Scope
  Sign : Signum
  Square1 : Math  Operator=square
  Trigonometric Function1 : Trigonometry
  Fx : Outport
  wires:
  Beta/1 -> Scope2/1, Trigonometric Function1/1, Modulo by Constant/1
  Product3/1 -> Product2/2
  Compare To Constant1/1 -> Logical Operator/2
  Compare To Constant/1 -> Logical Operator/1
  Gain3/1 -> Product2/1
  Trigonometric Function1/1 -> Product3/2
  Square1/1 -> Gain3/1
  Modulo by Constant/1 -> Compare To Constant1/1, Compare To Constant/1
  dX/dt/1 -> Square1/1, Sign/1, Scope1/1
  Product2/1 -> Scope/1, Fx/1
  Constant1/1 -> Product3/1
  Sign/1 -> Gain/1
  Gain/1 -> Product2/3
  Logical Operator/1 -> Product2/4

== system model2/Effet parasite sur fuselage/changement repère 1//1 ==
  y1 : Inport
  x1 : Inport  Port=2
  Beta : Inport  Port=3
  Product{,1..3} (4 alike) : Product
  Sum1 : Sum  Inputs=|-+
  Sum2 : Sum  Inputs=|++
  Trigonometric Function : Trigonometry
  Trigonometric Function1 : Trigonometry  Operator=cos
  y : Outport
  x : Outport  Port=2
  wires:
  Beta/1 -> Trigonometric Function1/1, Trigonometric Function/1
  Trigonometric Function/1 -> Product3/1, Product2/1
  Product2/1 -> Sum1/1
  y1/1 -> Product/2, Product2/2
  x1/1 -> Product3/2, Product1/2
  Trigonometric Function1/1 -> Product/1, Product1/1
  Product1/1 -> Sum1/2
  Sum1/1 -> x/1
  Product3/1 -> Sum2/2
  Product/1 -> Sum2/1
  Sum2/1 -> y/1

== system model2/Effort aéro/changement repère 1//1 ==
  y1 : Inport
  x1 : Inport  Port=2
  Beta : Inport  Port=3
  Product{,1..3} (4 alike) : Product
  Sum1 : Sum  Inputs=|-+
  Sum2 : Sum  Inputs=|++
  Trigonometric Function : Trigonometry
  Trigonometric Function1 : Trigonometry  Operator=cos
  y : Outport
  x : Outport  Port=2
  wires:
  Beta/1 -> Trigonometric Function1/1, Trigonometric Function/1
  Trigonometric Function/1 -> Product3/1, Product2/1
  Product2/1 -> Sum1/1
  y1/1 -> Product/2, Product2/2
  x1/1 -> Product3/2, Product1/2
  Trigonometric Function1/1 -> Product/1, Product1/1
  Product1/1 -> Sum1/2
  Sum1/1 -> x/1
  Product3/1 -> Sum2/2
  Product/1 -> Sum2/1
  Sum2/1 -> y/1

== system model2/Pivot moteur/changement repère 1//1 ==
  y1 : Inport
  x1 : Inport  Port=2
  Beta : Inport  Port=3
  Product{,1..3} (4 alike) : Product
  Sum1 : Sum  Inputs=|-+
  Sum2 : Sum  Inputs=|++
  Trigonometric Function : Trigonometry
  Trigonometric Function1 : Trigonometry  Operator=cos
  y : Outport
  x : Outport  Port=2
  wires:
  Beta/1 -> Trigonometric Function1/1, Trigonometric Function/1
  Trigonometric Function/1 -> Product3/1, Product2/1
  Product2/1 -> Sum1/1
  y1/1 -> Product/2, Product2/2
  x1/1 -> Product3/2, Product1/2
  Trigonometric Function1/1 -> Product/1, Product1/1
  Product1/1 -> Sum1/2
  Sum1/1 -> x/1
  Product3/1 -> Sum2/2
  Product/1 -> Sum2/1
  Sum2/1 -> y/1

== system model2/Pivot moteur/changement repère inverse2//1 ==
  y2 : Inport
  x2 : Inport  Port=2
  theta : Inport  Port=3
  Product{,1..3} (4 alike) : Product
  Sum1 : Sum  Inputs=|-+
  Sum2 : Sum  Inputs=|++
  Trigonometric Function : Trigonometry
  Trigonometric Function1 : Trigonometry  Operator=cos
  x1 : Outport
  y1 : Outport  Port=2
  wires:
  theta/1 -> Trigonometric Function1/1, Trigonometric Function/1
  Trigonometric Function/1 -> Product3/1, Product2/1
  Product2/1 -> Sum1/1
  Trigonometric Function1/1 -> Product/1, Product1/1
  Product1/1 -> Sum1/2
  Sum1/1 -> y1/1
  Product3/1 -> Sum2/2
  Product/1 -> Sum2/1
  Sum2/1 -> x1/1
  x2/1 -> Product/2, Product2/2
  y2/1 -> Product1/2, Product3/2
